simulink model "Standalone_CurrentControl"  (R2023b)
settings: Solver=FixedStepAuto  StartTime=0.0  StopTime=Inf  RelTol=1e-3  EnableMultiTasking=on
undefined symbols (not defined in the file): ControlCurrentPID_I, ControlCurrentPID_P, ControlInverter_DCVoltage, ControlPWM_PercentAtZeroVolt, ControlPWM_PercentPerVolt, SensorCurrent_VoltAtZero, SensorCurrent_VoltPerAmp, SimulationElectrical_Timestep
libraries: mcbcontrolslib x6, slpidlib x2
settings Model: DataDictionary=Data_GeneralDefinition.sldd  SimulationMode=external  ExtModeTrigDuration=20  Creator=rodri  LastModifiedBy=rodri
settings OptimizationCC: DefaultUnderspecifiedDataType=single  EnhancedBackFolding=on  PassReuseOutputArgsAs=Individual arguments  MaxStackSize=1024  OptimizeBlockOrder=speed  DifferentSizesBufferReuse=on  EfficientTunableParamExpr=on
settings DebuggingCC: ParameterTunabilityLossMsg=error
settings HardwareCC: ProdBitPerChar=16  ProdBitPerInt=16  ProdBitPerPointer=32  ProdBitPerSizeT=32  ProdBitPerPtrDiffT=32  ProdLargestAtomicInteger=Integer  ProdLargestAtomicFloat=None  ProdWordSize=16  ProdLongLongMode=on  ProdHWDeviceType=Texas Instruments->C2000  HardwareBoardFeatureSet=SoCBlockset
settings ModelReferenceCC: ModelReferenceNumInstancesAllowed=Single
settings SFSimCC: MATLABDynamicMemAlloc=off
settings RTWCC: Description=Embedded Coder  SystemTargetFile=ert.tlc  HardwareBoard=TI Piccolo F28069M LaunchPad  TemplateMakefile=ert_default_tmf  Toolchain=Texas Instruments Code Composer Studio (C2000)  CodeProfilingSaveOptions=MetricsOnly
settings CodeAppCC: ForceParamTrailComments=on  IgnoreCustomStorageClasses=off  OperatorAnnotations=on  SimulinkDataObjDesc=on  SFDataObjDesc=on  InsertBlockDesc=on
settings ERTTargetCC: CodeReplacementLibrary=TI C28x  ExtMode=on  ExtModeTransport=4  ExtModeStaticAlloc=on  ExtModeAutomaticAllocSize=off  ExtModeStaticAllocSize=2000  ExtModeMexFile=ext_xcp  ExtModeMexArgs=1 4 115200  ExtModeIntrfLevel=Level2 - Open

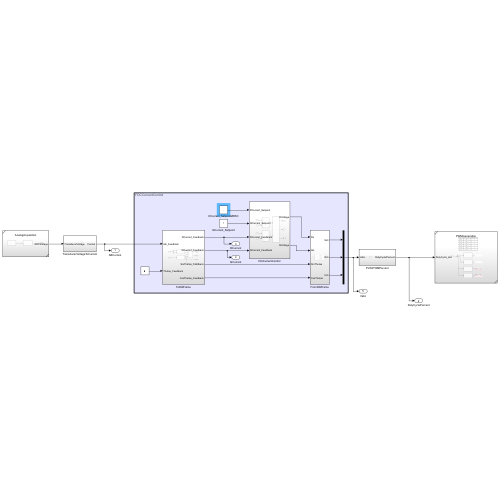
[thumbnail: Simulink's stored preview of the top-level diagram]
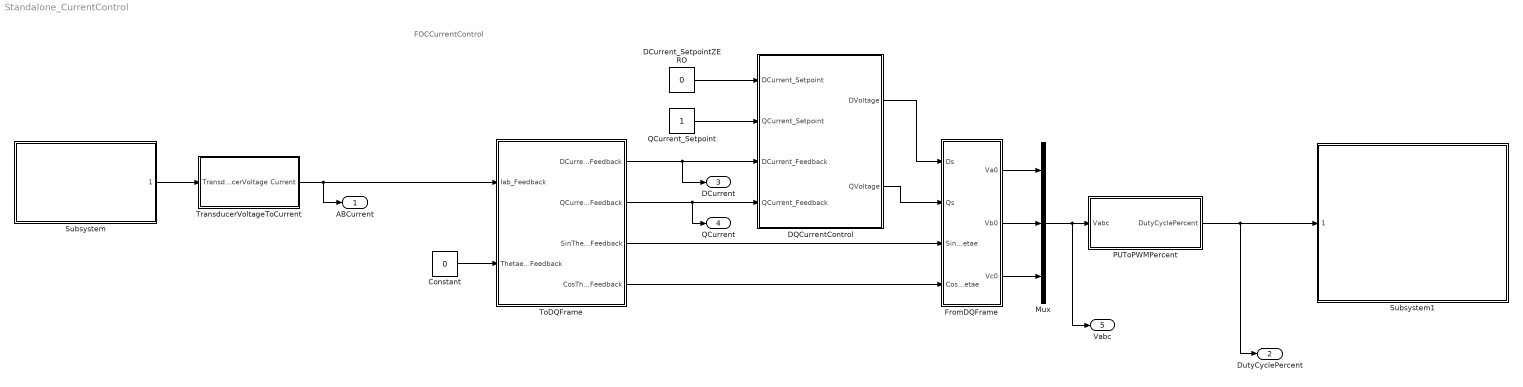
== system Standalone_CurrentControl ==
  note: FOCCurrentControl
  Constant : Constant  Value=0
  DCurrent_SetpointZERO : Constant  Value=0
  DQCurrentControl : Subsystem
  FromDQFrame : Subsystem
  Mux : Mux  Inputs=3
  PUToPWMPercent : Subsystem
  QCurrent_Setpoint : Constant
  Subsystem : Subsystem  ReferencedSubsystem=AnalogAcquisition
  Subsystem1 : Subsystem  ReferencedSubsystem=PWMGeneration
  ToDQFrame : Subsystem
  TransducerVoltageToCurrent : Subsystem
  ABCurrent : Outport
  DutyCyclePercent : Outport  Port=2
  DCurrent : Outport  Port=3
  QCurrent : Outport  Port=4
  Vabc : Outport  Port=5
  wires:
  Subsystem/1 -> TransducerVoltageToCurrent/1(TransducerVoltage)
  Mux/1 -> Vabc/1, PUToPWMPercent/1(Vabc)
  PUToPWMPercent/1(DutyCyclePercent) -> Subsystem1/1, DutyCyclePercent/1
  FromDQFrame/3(Vc0) -> Mux/3
  FromDQFrame/2(Vb0) -> Mux/2
  FromDQFrame/1(Va0) -> Mux/1
  DQCurrentControl/2(QVoltage) -> FromDQFrame/2(Qs)
  DQCurrentControl/1(DVoltage) -> FromDQFrame/1(Ds)
  ToDQFrame/2(QCurrent_Feedback) -> QCurrent/1, DQCurrentControl/4(QCurrent_Feedback)
  ToDQFrame/1(DCurrent_Feedback) -> DCurrent/1, DQCurrentControl/3(DCurrent_Feedback)
  Constant/1 -> ToDQFrame/2(Thetae_Feedback)
  DCurrent_SetpointZERO/1 -> DQCurrentControl/1(DCurrent_Setpoint)
  ToDQFrame/3(SinThetae_Feedback) -> FromDQFrame/3(SinThetae)
  TransducerVoltageToCurrent/1(Current) -> ToDQFrame/1(Iab_Feedback), ABCurrent/1
  QCurrent_Setpoint/1 -> DQCurrentControl/2(QCurrent_Setpoint)
  ToDQFrame/4(CosThetae_Feedback) -> FromDQFrame/4(CosThetae)

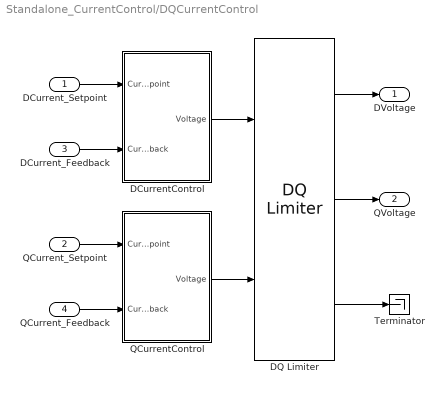
== system Standalone_CurrentControl/DQCurrentControl ==
  DCurrent_Setpoint : Inport
  QCurrent_Setpoint : Inport  Port=2
  DCurrent_Feedback : Inport  Port=3
  QCurrent_Feedback : Inport  Port=4
  DCurrentControl : Subsystem
  DQ Limiter : mcbcontrolslib/DQ Limiter  satMethodInputType=Specify via dialog  satMethodSelected=D-Q equivalence  satLimitInputType=Specify via dialog  Vmax=0.56*ControlInverter_DCVoltage
      settings: LibrarySourceBlock=mcbhdllib/Controls/Control Reference/DQ Limiter
  QCurrentControl : Subsystem
  Terminator : Terminator
  DVoltage : Outport
  QVoltage : Outport  Port=2
  wires:
  DCurrent_Feedback/1 -> DCurrentControl/2(Current_Feedback)
  QCurrent_Feedback/1 -> QCurrentControl/2(Current_Feedback)
  QCurrent_Setpoint/1 -> QCurrentControl/1(Current_Setpoint)
  DCurrentControl/1(Voltage) -> DQ Limiter/1
  QCurrentControl/1(Voltage) -> DQ Limiter/2
  DCurrent_Setpoint/1 -> DCurrentControl/1(Current_Setpoint)
  DQ Limiter/1 -> DVoltage/1
  DQ Limiter/2 -> QVoltage/1
  DQ Limiter/3 -> Terminator/1

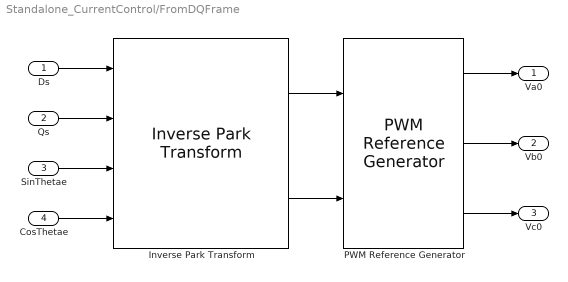
== system Standalone_CurrentControl/FromDQFrame ==
  Ds : Inport
  Qs : Inport  Port=2
  SinThetae : Inport  Port=3
  CosThetae : Inport  Port=4
  Inverse Park Transform : mcbcontrolslib/Inverse Park Transform  PhaseInput=Two inputs  AxisAlignment=D-axis  ThetaInput=Sine and Cosine electrical position  AngleInput=Per-unit  N_points=1024
      settings: LibrarySourceBlock=mcbhdllib/Controls/Math Transforms/Inverse Park Transform
  PWM Reference Generator : mcbcontrolslib/PWM Reference Generator  inSignal=Valphabeta  modType=SPWM: sinusoidal PWM
      settings: LibrarySourceBlock=mcblib/Controls/Math Transforms/PWM Reference Generator
  Va0 : Outport
  Vb0 : Outport  Port=2
  Vc0 : Outport  Port=3
  wires:
  Inverse Park Transform/1 -> PWM Reference Generator/1
  Qs/1 -> Inverse Park Transform/2
  Inverse Park Transform/2 -> PWM Reference Generator/2
  PWM Reference Generator/3 -> Vc0/1
  PWM Reference Generator/2 -> Vb0/1
  PWM Reference Generator/1 -> Va0/1
  CosThetae/1 -> Inverse Park Transform/4
  Ds/1 -> Inverse Park Transform/1
  SinThetae/1 -> Inverse Park Transform/3

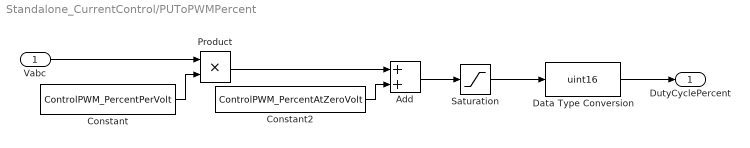
== system Standalone_CurrentControl/PUToPWMPercent ==
  Vabc : Inport
  Add : Sum
  Constant : Constant  Value=ControlPWM_PercentPerVolt  OutDataTypeStr=Inherit: Inherit via back propagation  SampleTime=-1
  Constant2 : Constant  Value=ControlPWM_PercentAtZeroVolt  OutDataTypeStr=Inherit: Inherit via back propagation  SampleTime=-1
  Data Type Conversion : DataTypeConversion  OutDataTypeStr=uint16  SaturateOnIntegerOverflow=off  RndMeth=Floor
  Product : Product  OutDataTypeStr=Inherit: Inherit via back propagation
  Saturation : Saturate  UpperLimit=100  LowerLimit=0
  DutyCyclePercent : Outport
  wires:
  Vabc/1 -> Product/1
  Add/1 -> Saturation/1
  Constant/1 -> Product/2
  Product/1 -> Add/1
  Constant2/1 -> Add/2
  Saturation/1 -> Data Type Conversion/1
  Data Type Conversion/1 -> DutyCyclePercent/1

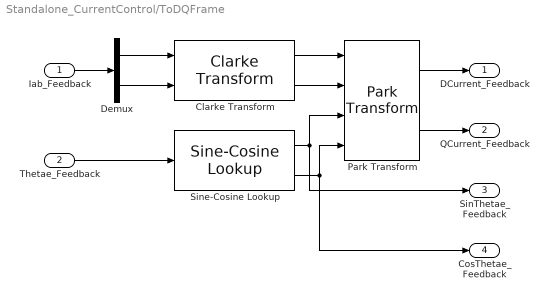
== system Standalone_CurrentControl/ToDQFrame ==
  Iab_Feedback : Inport
  Thetae_Feedback : Inport  Port=2
  Clarke Transform : mcbcontrolslib/Clarke Transform  VariantControl=Variant2  PhaseInput=Two inputs  EnPowerInv=off
      settings: LibrarySourceBlock=mcbhdllib/Controls/Math Transforms/Clarke Transform
  Demux : Demux  Outputs=2
  Park Transform : mcbcontrolslib/Park Transform  PhaseInput=Two inputs  AxisAlignment=D-axis  ThetaInput=Sine and Cosine electrical position  AngleInput=Per-unit  N_points=1024
      settings: LibrarySourceBlock=mcbhdllib/Controls/Math Transforms/Park Transform
  Sine-Cosine Lookup : mcbcontrolslib/Sine-Cosine Lookup  AngleInput=Radians  N_points=1024
      settings: LibrarySourceBlock=mcblib/Controls/Math Transforms/Sine-Cosine Lookup
  DCurrent_Feedback : Outport
  QCurrent_Feedback : Outport  Port=2
  SinThetae_Feedback : Outport  Port=3
  CosThetae_Feedback : Outport  Port=4
  wires:
  Clarke Transform/1 -> Park Transform/1
  Demux/2 -> Clarke Transform/2
  Clarke Transform/2 -> Park Transform/2
  Park Transform/2 -> QCurrent_Feedback/1
  Demux/1 -> Clarke Transform/1
  Sine-Cosine Lookup/1 -> Park Transform/3, SinThetae_Feedback/1
  Park Transform/1 -> DCurrent_Feedback/1
  Sine-Cosine Lookup/2 -> Park Transform/4, CosThetae_Feedback/1
  Thetae_Feedback/1 -> Sine-Cosine Lookup/1
  Iab_Feedback/1 -> Demux/1

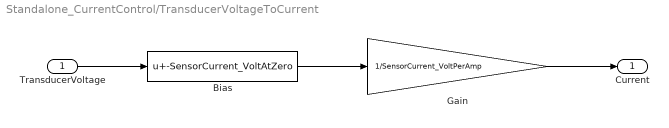
== system Standalone_CurrentControl/TransducerVoltageToCurrent ==
  TransducerVoltage : Inport
  Bias : Bias  Bias=-SensorCurrent_VoltAtZero  SaturateOnIntegerOverflow=off
  Gain : Gain  Gain=1/SensorCurrent_VoltPerAmp
  Current : Outport
  wires:
  Gain/1 -> Current/1
  TransducerVoltage/1 -> Bias/1
  Bias/1 -> Gain/1

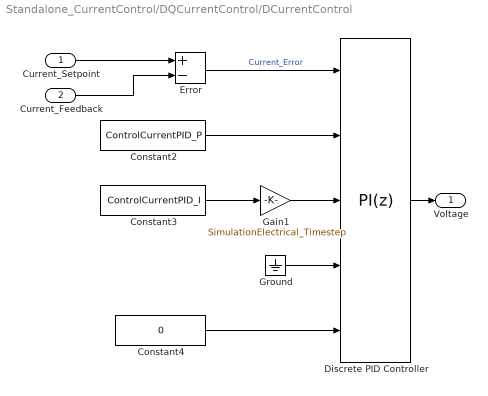
== system Standalone_CurrentControl/DQCurrentControl/DCurrentControl ==
  Current_Setpoint : Inport
  Current_Feedback : Inport  Port=2
  Constant2 : Constant  Value=ControlCurrentPID_P  SampleTime=-1
  Constant3 : Constant  Value=ControlCurrentPID_I  SampleTime=-1
  Constant4 : Constant  Value=0  OutDataTypeStr=Inherit: Inherit via back propagation  SampleTime=-1
  Discrete PID Controller : slpidlib/PID Controller  Controller=PI  Form=Parallel  TimeDomain=Discrete-time  UseExternalTs=off  SampleTime=-1  IntegratorMethod=Forward Euler  FilterMethod=Forward Euler  ControllerParametersSource=external  P=ControlCurrentPID_P  I=ControlCurrentPID_I*SimulationElectrical_Timestep  UseKiTs=on  D=0  N=100  UseFilter=on  TunerSelectOption=Transfer Function Based (PID Tuner App)  InitialConditionSource=external  InitialConditionForIntegrator=0  InitialConditionForFilter=0  DifferentiatorICPrevScaledInput=0  ExternalReset=level  TrackingMode=off  Kt=1  LimitOutput=on  SatLimitsSource=internal  UpperSaturationLimit=0.56*ControlInverter_DCVoltage  LowerSaturationLimit=-0.56*ControlInverter_DCVoltage  LinearizeAsGain=off  AntiWindupMode=clamping  Kb=1  LimitIntegrator=off  UpperIntegratorSaturationLimit=inf  LowerIntegratorSaturationLimit=-inf  RndMeth=Simplest  POutMin=[]  POutMax=[]  IOutMin=[]  IOutMax=[]  DOutMin=[]  DOutMax=[]  NOutMin=[]  NOutMax=[]  SumOutMin=[]  SumOutMax=[]  SaturationOutDataTypeStr=Inherit: Inherit via back propagation  SaturationOutMin=[]  SaturationOutMax=[]  PParamMin=[]  PParamMax=[]  IParamMin=[]  IParamMax=[]  DParamMin=[]  DParamMax=[]  NParamMin=[]  NParamMax=[]  KbParamMin=[]  KbParamMax=[]  KtParamMin=[]  KtParamMax=[]  KbOutMin=[]  KbOutMax=[]  KtOutMin=[]  KtOutMax=[]  IntegratorOutMin=[]  IntegratorOutMax=[]  FilterOutMin=[]  FilterOutMax=[]  SumI1OutMin=[]  SumI1OutMax=[]  SumI2OutMin=[]  SumI2OutMax=[]  SumI3OutMin=[]  SumI3OutMax=[]  SumI4OutMin=[]  SumI4OutMax=[]  SumDOutMin=[]  SumDOutMax=[]  DifferentiatorOutMin=[]  DifferentiatorOutMax=[]  FilterDiffOutCoefMin=[]  FilterDiffOutCoefMax=[]  ReciprocalOutMin=[]  ReciprocalOutMax=[]  SumDenOutMin=[]  SumDenOutMax=[]  SumNumOutMin=[]  SumNumOutMax=[]  DivideOutMin=[]  DivideOutMax=[]  UdiffTsProdOutMin=[]  UdiffTsProdOutMax=[]  NTsProdOutMin=[]  NTsProdOutMax=[]  UintegralTsProdOutMin=[]  UintegralTsProdOutMax=[]  UngainTsProdOutMin=[]  UngainTsProdOutMax=[]  ClampingZeroOutDataTypeStr=Inherit: Inherit via back propagation  ClampingZeroOutMin=[]  ClampingZeroOutMax=[]  FilterDenConstantOutDataTypeStr=Inherit: Inherit via back propagation  FilterDenConstantOutMin=[]  FilterDenConstantOutMax=[]  PCopyOutDataTypeStr=Inherit: Inherit via back propagation  PCopyOutMin=[]  PCopyOutMax=[]  NCopyOutDataTypeStr=Inherit: Inherit via back propagation  NCopyOutMin=[]  NCopyOutMax=[]  IntegratorContinuousStateAttributes=''  IntegratorStateMustResolveToSignalObject=off  IntegratorRTWStateStorageClass=Auto  FilterContinuousStateAttributes=''  FilterStateMustResolveToSignalObject=off  FilterRTWStateStorageClass=Auto  ParallelPVariant=ExternalParameters  IdealPVariant=Disabled  IVariant=ExternalParameters  DVariant=Disabled  IntegratorVariant=Discrete  SatVariant=Enabled  AWVariant=DiscClampingParallel  PCopyVariant=Disabled  TRVariant=Disabled  FdbkBlocksVariant=Forward  IdealPFdbkVariant=Disabled  SatFdbkVariant=Disabled  DerivativeFilterVariant=Disabled  NVariant=Disabled  NCopyVariant=Disabled_SignalSpec  FilterICVariant=Disabled  IntegratorICVariant=ExternalICs  ExternalResetVariant=ExternalReset  TRSumVariant=Passthrough  SumFdbkVariant=Disabled  SumVariant=Sum_PI  TsampFilterVariant=InternalTs  TsampNgainVariant=Passthrough  TsampIntegralVariant=Disabled_SignalSpec  ExternalSaturationOutDataTypeStr=Inherit: Same as second input
      settings: LibrarySourceBlock=simulink/Discrete/Discrete PID Controller
  Error : Sum  Inputs=+-
  Gain1 : Gain  Gain=SimulationElectrical_Timestep
  Ground : Ground
  Voltage : Outport
  wires:
  Constant2/1 -> Discrete PID Controller/2
  Constant4/1 -> Discrete PID Controller/5
  Discrete PID Controller/1 -> Voltage/1
  Error/1 -> Discrete PID Controller/1  "Current_Error"
  Current_Setpoint/1 -> Error/1
  Constant3/1 -> Gain1/1
  Gain1/1 -> Discrete PID Controller/3
  Ground/1 -> Discrete PID Controller/4
  Current_Feedback/1 -> Error/2

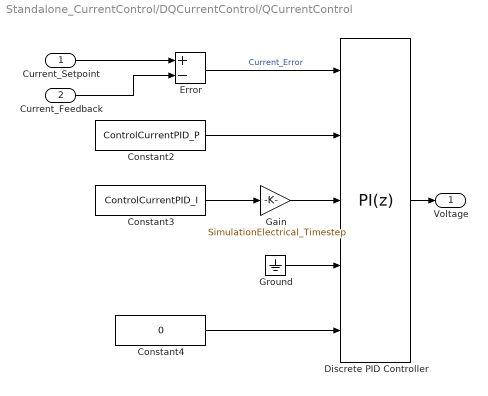
== system Standalone_CurrentControl/DQCurrentControl/QCurrentControl ==
  Current_Setpoint : Inport
  Current_Feedback : Inport  Port=2
  Constant2 : Constant  Value=ControlCurrentPID_P  OutDataTypeStr=Inherit: Inherit via back propagation
  Constant3 : Constant  Value=ControlCurrentPID_I  OutDataTypeStr=Inherit: Inherit via back propagation
  Constant4 : Constant  Value=0  OutDataTypeStr=Inherit: Inherit via back propagation
  Discrete PID Controller : slpidlib/PID Controller  Controller=PI  Form=Parallel  TimeDomain=Discrete-time  UseExternalTs=off  SampleTime=-1  IntegratorMethod=Forward Euler  FilterMethod=Forward Euler  ControllerParametersSource=external  P=ControlCurrentPID_P  I=ControlCurrentPID_I*SimulationElectrical_Timestep  UseKiTs=on  D=0  N=100  UseFilter=on  TunerSelectOption=Transfer Function Based (PID Tuner App)  InitialConditionSource=external  InitialConditionForIntegrator=0  InitialConditionForFilter=0  DifferentiatorICPrevScaledInput=0  ExternalReset=level  TrackingMode=off  Kt=1  LimitOutput=on  SatLimitsSource=internal  UpperSaturationLimit=0.56*ControlInverter_DCVoltage  LowerSaturationLimit=-0.56*ControlInverter_DCVoltage  LinearizeAsGain=off  AntiWindupMode=clamping  Kb=1  LimitIntegrator=off  UpperIntegratorSaturationLimit=inf  LowerIntegratorSaturationLimit=-inf  POutMin=[]  POutMax=[]  IOutMin=[]  IOutMax=[]  DOutMin=[]  DOutMax=[]  NOutMin=[]  NOutMax=[]  SumOutMin=[]  SumOutMax=[]  SaturationOutDataTypeStr=Inherit: Inherit via back propagation  SaturationOutMin=[]  SaturationOutMax=[]  PParamMin=[]  PParamMax=[]  IParamMin=[]  IParamMax=[]  DParamMin=[]  DParamMax=[]  NParamMin=[]  NParamMax=[]  KbParamMin=[]  KbParamMax=[]  KtParamMin=[]  KtParamMax=[]  KbOutMin=[]  KbOutMax=[]  KtOutMin=[]  KtOutMax=[]  IntegratorOutMin=[]  IntegratorOutMax=[]  FilterOutMin=[]  FilterOutMax=[]  SumI1OutMin=[]  SumI1OutMax=[]  SumI2OutMin=[]  SumI2OutMax=[]  SumI3OutMin=[]  SumI3OutMax=[]  SumI4OutMin=[]  SumI4OutMax=[]  SumDOutMin=[]  SumDOutMax=[]  DifferentiatorOutMin=[]  DifferentiatorOutMax=[]  FilterDiffOutCoefMin=[]  FilterDiffOutCoefMax=[]  ReciprocalOutMin=[]  ReciprocalOutMax=[]  SumDenOutMin=[]  SumDenOutMax=[]  SumNumOutMin=[]  SumNumOutMax=[]  DivideOutMin=[]  DivideOutMax=[]  UdiffTsProdOutMin=[]  UdiffTsProdOutMax=[]  NTsProdOutMin=[]  NTsProdOutMax=[]  UintegralTsProdOutMin=[]  UintegralTsProdOutMax=[]  UngainTsProdOutMin=[]  UngainTsProdOutMax=[]  ClampingZeroOutDataTypeStr=Inherit: Inherit via back propagation  ClampingZeroOutMin=[]  ClampingZeroOutMax=[]  FilterDenConstantOutDataTypeStr=Inherit: Inherit via back propagation  FilterDenConstantOutMin=[]  FilterDenConstantOutMax=[]  PCopyOutDataTypeStr=Inherit: Inherit via back propagation  PCopyOutMin=[]  PCopyOutMax=[]  NCopyOutDataTypeStr=Inherit: Inherit via back propagation  NCopyOutMin=[]  NCopyOutMax=[]  IntegratorContinuousStateAttributes=''  IntegratorStateMustResolveToSignalObject=off  IntegratorRTWStateStorageClass=Auto  FilterContinuousStateAttributes=''  FilterStateMustResolveToSignalObject=off  FilterRTWStateStorageClass=Auto  ParallelPVariant=ExternalParameters  IdealPVariant=Disabled  IVariant=ExternalParameters  DVariant=Disabled  IntegratorVariant=Discrete  SatVariant=Enabled  AWVariant=DiscClampingParallel  PCopyVariant=Disabled  TRVariant=Disabled  FdbkBlocksVariant=Forward  IdealPFdbkVariant=Disabled  SatFdbkVariant=Disabled  DerivativeFilterVariant=Disabled  NVariant=Disabled  NCopyVariant=Disabled_SignalSpec  FilterICVariant=Disabled  IntegratorICVariant=ExternalICs  ExternalResetVariant=ExternalReset  TRSumVariant=Passthrough  SumFdbkVariant=Disabled  SumVariant=Sum_PI  TsampFilterVariant=InternalTs  TsampNgainVariant=Passthrough  TsampIntegralVariant=Disabled_SignalSpec  ExternalSaturationOutDataTypeStr=Inherit: Same as second input
      settings: LibrarySourceBlock=simulink/Discrete/Discrete PID Controller
  Error : Sum  Inputs=+-
  Gain : Gain  Gain=SimulationElectrical_Timestep
  Ground : Ground
  Voltage : Outport
  wires:
  Current_Feedback/1 -> Error/2
  Ground/1 -> Discrete PID Controller/4
  Constant3/1 -> Gain/1
  Current_Setpoint/1 -> Error/1
  Error/1 -> Discrete PID Controller/1  "Current_Error"
  Discrete PID Controller/1 -> Voltage/1
  Constant4/1 -> Discrete PID Controller/5
  Gain/1 -> Discrete PID Controller/3
  Constant2/1 -> Discrete PID Controller/2
